simulink model "nmsRR"  (R2021a)
settings: Solver=ode15s  StartTime=0.0  StopTime=t  MaxStep=1e-2  RelTol=1e-2
StartFcn:
  | tic
StopFcn:
  | toc
  | 
  | 
  | %if GimbalLockFlag
  |  % fprintf(2, 'Almost reached Gimbal Lock of IMU. Simulation stopped.\n')
  | %end
  | 
  | %fprintf('Elapsed time: %4.2f sec (%4.2f%% realtime)\n', a, tout(end)/a*100)
undefined symbols (not defined in the file): Balance02, Balance13, BalanceTrunk, BasisStim, CompensateSwing, CompliantLeg, FlexAnkle, Ground, ICs, init_des_left, init_des_right, init_l_left, init_l_right, init_q_del, init_sensor_body, init_sensor_world, init_v_left, init_v_right, LateralControl, mParams, PreventKneeOverextension, StepDur, Target02, Target13, theta0, X, Y, Z
libraries: simulink_extras x133, nesl_utility x105, sm_lib x88, simulink x72, robotcorelib x5, dspinverses x5, dspswit3 x2, vrlib x2, robotmaniplib x1
(part 3 of 8)

== system nmsRR/CMA Data/check steady state ==
  p : Inport
  nStep : Inport  Port=2
  Abs : Abs  ZeroCross=off
  Add{,1..9,15..16} (12 alike) : Sum  Inputs=-+
  Add{10..14,17} (6 alike) : Sum  Inputs=+-
  Demux2 : Demux  Outputs=7
  Demux3 : Demux  Outputs=7
  Fcn : Fcn  Expr=rem(u(1), 2)
  Gain14 : Gain  Gain=.5
  Mux1 : Mux  Inputs=6
  Rounding Function1 : Rounding
  Scope : Scope
  Sum of Elements : Sum  Inputs=+
  even : Subsystem  TreatAsAtomicUnit=on
  odd : Subsystem  TreatAsAtomicUnit=on
  SS_dist : Outport  VectorParamsAs1DForOutWhenUnconnected=off
  wires:
  p/1 -> even/1(In1), odd/1(In1)
  Fcn/1 -> odd/Trigger, even/Trigger
  odd/1(Out1) -> Scope/1, Demux2/1
  even/1(Out1) -> Demux3/1
  Add10/1 -> Mux1/1
  Add11/1 -> Mux1/2
  Add12/1 -> Mux1/3
  Add13/1 -> Mux1/4
  Add14/1 -> Mux1/5
  Demux2/2 -> Add/2
  Demux2/3 -> Add1/2
  Demux2/4 -> Add2/2
  Demux2/5 -> Add3/2
  Demux2/6 -> Add4/2
  Demux2/1 -> Add/1, Add1/1, Add2/1, Add3/1, Add4/1, Add15/1
  Demux3/2 -> Add5/2
  Demux3/3 -> Add6/2
  Demux3/4 -> Add7/2
  Demux3/5 -> Add8/2
  Demux3/6 -> Add9/2
  Demux3/1 -> Add5/1, Add6/1, Add7/1, Add8/1, Add9/1, Add16/1
  Add/1 -> Add10/1
  Add1/1 -> Add11/1
  Add2/1 -> Add12/1
  Add3/1 -> Add13/1
  Add4/1 -> Add14/1
  Add5/1 -> Add10/2
  Add6/1 -> Add11/2
  Add7/1 -> Add12/2
  Add8/1 -> Add13/2
  Add9/1 -> Add14/2
  Mux1/1 -> Abs/1
  Abs/1 -> Sum of Elements/1
  Sum of Elements/1 -> SS_dist/1
  nStep/1 -> Gain14/1
  Gain14/1 -> Rounding Function1/1
  Rounding Function1/1 -> Fcn/1
  Demux2/7 -> Add15/2
  Demux3/7 -> Add16/2
  Add15/1 -> Add17/1
  Add16/1 -> Add17/2
  Add17/1 -> Mux1/6

== system nmsRR/Muscle Actuation Layer/Muscles Left ==
  STIM Left : Inport
  Demux : Demux
  Muscle Dynamics (Vectorized)1 : Subsystem
  Muscle Length Vector1 : Subsystem
  Muscle Torque Contributions1 : Subsystem
  Scope : Scope
  Terminator : Terminator
  Terminator1 : Terminator
  tauHipPitchL : Outport
  tauHipRollL : Outport  Port=2
  tauKneeL : Outport  Port=3
  tauHipAnkleL : Outport  Port=4
  tag scope: LFmVec=global, LLceVec=global, LVceVec=global
  wires:
  Demux/2 -> Muscle Length Vector1/2(qHipRoll [rad])
  Muscle Torque Contributions1/2(tauHR [Nm]) -> tauHipRollL/1
  Demux/1 -> Muscle Length Vector1/1(qHipPitch [rad])
  Muscle Dynamics (Vectorized)1/1(Fmtc) -> Scope/1, Muscle Torque Contributions1/3(FmVec [N x11]), [LFmVec]
  Demux/4 -> Muscle Torque Contributions1/2(qAnkle [rad]), Muscle Length Vector1/4(qAnkle [rad])  "qA"
  Muscle Dynamics (Vectorized)1/3(Vce) -> [LVceVec]
  Muscle Torque Contributions1/3(tauK [Nm]) -> tauKneeL/1
  Demux/3 -> Muscle Torque Contributions1/1(qKnee [rad]), Muscle Length Vector1/3(qKnee [rad])  "qK"
  Muscle Dynamics (Vectorized)1/5(ForceLengthFactor) -> Terminator1/1
  Muscle Length Vector1/1(lmtc [m x11]) -> Muscle Dynamics (Vectorized)1/1(lmtc [m])
  Muscle Torque Contributions1/1(tauHP [Nm]) -> tauHipPitchL/1
  Muscle Torque Contributions1/4(tauA [Nm]) -> tauHipAnkleL/1
  Muscle Dynamics (Vectorized)1/4(A) -> Terminator/1
  Muscle Dynamics (Vectorized)1/2(Lce) -> [LLceVec]
  STIM Left/1 -> Muscle Dynamics (Vectorized)1/2(STIM)
  [Llegq] -> Demux/1

== system nmsRR/Muscle Actuation Layer/Muscles Right ==
  STIM Right : Inport
  Demux : Demux
  Goto15 : Goto  Commented=on  GotoTag=activation_R  TagVisibility=global
  Muscle Dynamics (Vectorized) : Subsystem
  Muscle Length Vector : Subsystem
  Muscle Torque Contributions : Subsystem
  R Leg Muscles Vce [m/s x11]1 : Goto  Commented=on  GotoTag=RForceLength  TagVisibility=global
  tauHipPitchR : Outport
  tauHipRollR : Outport  Port=2
  tauKneeR : Outport  Port=3
  tauHipAnkleR : Outport  Port=4
  tag scope: RFmVec=global, RLceVec=global, RVceVec=global
  wires:
  Muscle Torque Contributions/4(tauA [Nm]) -> tauHipAnkleR/1
  Muscle Torque Contributions/3(tauK [Nm]) -> tauKneeR/1
  Muscle Length Vector/1(lmtc [m x11]) -> Muscle Dynamics (Vectorized)/1(lmtc [m])
  Demux/3 -> Muscle Torque Contributions/1(qKnee [rad]), Muscle Length Vector/3(qKnee [rad])  "qK"
  Demux/4 -> Muscle Torque Contributions/2(qAnkle [rad]), Muscle Length Vector/4(qAnkle [rad])  "qA"
  Muscle Dynamics (Vectorized)/2(Lce) -> [RLceVec]
  Muscle Torque Contributions/2(tauHR [Nm]) -> tauHipRollR/1
  Demux/1 -> Muscle Length Vector/1(qHipPitch [rad])  "qHP"
  Muscle Dynamics (Vectorized)/5(ForceLengthFactor) -> R Leg Muscles Vce [m/s x11]1/1
  Muscle Dynamics (Vectorized)/1(Fmtc) -> Muscle Torque Contributions/3(FmVec [N x11]), [RFmVec]
  Muscle Dynamics (Vectorized)/4(A) -> Goto15/1
  Muscle Dynamics (Vectorized)/3(Vce) -> [RVceVec]
  Muscle Torque Contributions/1(tauHP [Nm]) -> tauHipPitchR/1
  Demux/2 -> Muscle Length Vector/2(qHipRoll [rad])  "qHR"
  STIM Right/1 -> Muscle Dynamics (Vectorized)/2(STIM)
  [Rlegq] -> Demux/1  "qHP"

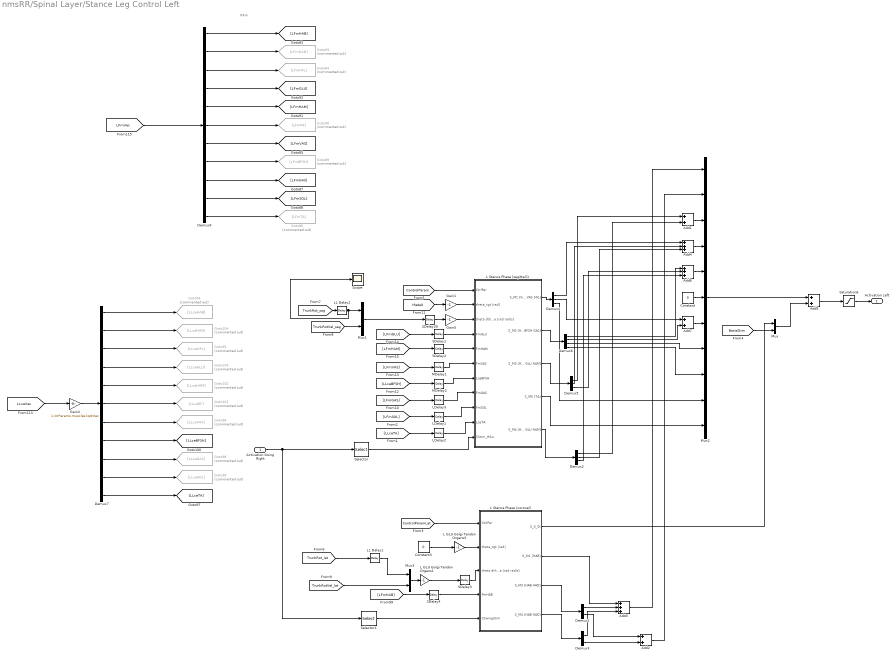
== system nmsRR/Spinal Layer/Stance Leg Control Left ==
  note: RFm
  Activation Swing Right : Inport
  Add{1..2,5,7} (4 alike) : Sum
  Add3 : Sum  Inputs=+++
  Add4 : Sum  Inputs=+++
  Add6 : Sum  Inputs=+++
  Constant : Constant  Value=0
  Constant3 : Constant  Value=0
  Demux1 : Demux  Outputs=2
  Demux2 : Demux  Outputs=3
  Demux3 : Demux  Outputs=2
  Demux4 : Demux  Outputs=3
  Demux5 : Demux  Outputs=3
  Demux6 : Demux
  Demux7 : Demux  Outputs=11
  Demux9 : Demux  Outputs=11
  Gain1 : Gain  Gain=-1
  Gain4 : Gain  Gain=1./mParams.muscles.loptVec
  Gain5 : Gain  Gain=-1
  Goto101 : Goto  Commented=on  GotoTag=LLceRF
  Goto102 : Goto  Commented=on  GotoTag=LLceHAM
  Goto103 : Goto  Commented=on  GotoTag=LLceGLU
  Goto104 : Goto  Commented=on  GotoTag=LLceHAD
  Goto84 : Goto  Commented=on  GotoTag=LFmHFL
  Goto86 : Goto  Commented=on  GotoTag=LFmTA
  Goto89 : Goto  Commented=on  GotoTag=LFmBFSH
  Goto90 : Goto  Commented=on  GotoTag=LFmRF
  Goto93 : Goto  Commented=on  GotoTag=LFmHAD
  Goto94 : Goto  Commented=on  GotoTag=LLceHAB
  Goto95 : Goto  Commented=on  GotoTag=LLceHFL
  Goto96 : Goto  Commented=on  GotoTag=LLceVAS
  Goto98 : Goto  Commented=on  GotoTag=LLceGAS
  Goto99 : Goto  Commented=on  GotoTag=LLceSOL
  L GLU Golgi Tendon Organs1 : Gain  Gain=-1
  L GLU Golgi Tendon Organs3 : Gain  Gain=-1
  L Stance Phase (coronal) : Subsystem  TreatAsAtomicUnit=on
  L Stance Phase (sagittal)1 : Subsystem  TreatAsAtomicUnit=on
  LDelay1 : TransportDelay  DelayTime=mParams.control.delays.long
  LDelay2 : TransportDelay  DelayTime=mParams.control.delays.long
  LDelay3 : TransportDelay  DelayTime=mParams.control.delays.long
  LL Delay1 : TransportDelay  DelayTime=mParams.control.delays.longloop/2
  LL Delay2 : TransportDelay  DelayTime=mParams.control.delays.longloop/2
  MDelay1 : TransportDelay  DelayTime=mParams.control.delays.mid
  MDelay2 : TransportDelay  DelayTime=mParams.control.delays.mid
  Mux : Mux  Inputs=2
  Mux1 : Mux  Inputs=2
  Mux2 : Mux  Inputs=11
  Mux3 : Mux  Inputs=2
  SDelay{1..4,29} (5 alike) : TransportDelay  DelayTime=mParams.control.delays.short
  Saturation6 : Saturate  UpperLimit=1  LowerLimit=0.01  ZeroCross=off
  Scope : Scope
  Selector : Selector  InputPortWidth=11  IndexOptions=Index vector (dialog)  Indices=[3 4 5 6]  OutputSizes=1
  Selector1 : Selector  InputPortWidth=11  IndexOptions=Index vector (dialog)  Indices=[1 2]  OutputSizes=1
  Activation Left : Outport
  wires:
  [LFmVec] -> Demux9/1
  Demux9/1 -> [LFmHAB]
  [ControlParam] -> L Stance Phase (sagittal)1/1(CtrlPar)
  Demux7/5 -> Goto102/1
  MDelay1/1 -> L Stance Phase (sagittal)1/6(FmVAS)
  Gain4/1 -> Demux7/1
  Demux9/5 -> [LFmHAM]
  Demux7/10 -> Goto99/1
  Demux7/8 -> [LLceBFSH]
  Mux1/1 -> SDelay29/1
  Demux7/3 -> Goto95/1
  Demux7/9 -> Goto98/1
  LDelay2/1 -> L Stance Phase (sagittal)1/10(LceTA)
  Demux9/3 -> Goto84/1
  LDelay1/1 -> L Stance Phase (sagittal)1/9(FmSOL)
  Demux9/11 -> Goto86/1
  [LLceVec] -> Gain4/1
  Demux9/9 -> [LFmGAS]
  Demux7/4 -> Goto103/1
  SDelay2/1 -> L Stance Phase (sagittal)1/5(FmHAM)
  Demux9/10 -> [LFmSOL]
  Gain5/1 -> L Stance Phase (sagittal)1/3(theta dtheta [rad rad/s])
  Demux7/2 -> Goto104/1
  Demux9/4 -> [LFmGLU]
  SDelay29/1 -> Gain5/1
  Demux9/6 -> Goto90/1
  Demux9/8 -> Goto89/1
  Demux9/7 -> [LFmVAS]
  Demux7/11 -> [LLceTA]
  LDelay3/1 -> L Stance Phase (sagittal)1/8(FmGAS)
  SDelay1/1 -> L Stance Phase (sagittal)1/4(FmGLU)
  Demux7/7 -> Goto96/1
  Demux7/1 -> Goto94/1
  Demux9/2 -> Goto93/1
  Demux7/6 -> Goto101/1
  MDelay2/1 -> L Stance Phase (sagittal)1/7(LceBFSH)
  Saturation6/1 -> Activation Left/1
  Add5/1 -> Saturation6/1
  Mux/1 -> Add5/2
  [theta0] -> Gain1/1
  Gain1/1 -> L Stance Phase (sagittal)1/2(theta_tgt [rad])
  [BasisStim] -> Mux/2
  [ControlParamLat] -> L Stance Phase (coronal)/1(CtrlPar)
  SDelay3/1 -> L Stance Phase (coronal)/3(theta dtheta [rad rad/s])
  [LFmHAB] -> SDelay4/1
  SDelay4/1 -> L Stance Phase (coronal)/4(FmHAB)
  L GLU Golgi Tendon Organs1/1 -> SDelay3/1
  L GLU Golgi Tendon Organs3/1 -> L Stance Phase (coronal)/2(theta_tgt [rad])
  Constant3/1 -> L GLU Golgi Tendon Organs3/1
  Mux3/1 -> L GLU Golgi Tendon Organs1/1
  L Stance Phase (coronal)/1(S_0_St) -> Mux/1
  L Stance Phase (coronal)/2(S_M1 [HAB]) -> Add3/1
  L Stance Phase (coronal)/3(S_M3 [HAB HAD]) -> Demux1/1
  Demux1/1 -> Add3/2
  [TrunkRot_sag] -> LL Delay2/1
  LL Delay2/1 -> Scope/1, Mux1/1
  [TrunkRotVel_sag] -> Mux1/2
  [TrunkRot_lat] -> LL Delay1/1
  LL Delay1/1 -> Mux3/1
  [TrunkRotVel_lat] -> Mux3/2
  [LFmGLU] -> SDelay1/1
  [LFmHAM] -> SDelay2/1
  [LFmVAS] -> MDelay1/1
  [LLceBFSH] -> MDelay2/1
  [LFmGAS] -> LDelay3/1
  [LFmSOL] -> LDelay1/1
  [LLceTA] -> LDelay2/1
  Demux4/3 -> Mux2/10
  Constant/1 -> Mux2/6
  L Stance Phase (sagittal)1/2(S_M2 [HAM VAS BFSH GAS]) -> Demux6/1
  Add6/1 -> Mux2/5
  Demux6/2 -> Add7/2
  Add4/1 -> Mux2/4
  Demux4/1 -> Add4/1
  Add3/1 -> Mux2/1
  Demux4/2 -> Add7/1
  Demux6/4 -> Mux2/9
  L Stance Phase (sagittal)1/4(S_M5 [TA]) -> Mux2/11
  Demux1/2 -> Add2/1
  Demux6/3 -> Mux2/8
  Mux2/1 -> Add5/1
  Add7/1 -> Mux2/7
  Demux6/1 -> Add6/1
  Demux5/1 -> Add1/1
  Demux5/2 -> Add4/2
  Demux5/3 -> Add6/2
  L Stance Phase (sagittal)1/1(S_M1 [GLU VAS SOL]) -> Demux4/1
  L Stance Phase (sagittal)1/3(S_M3 [HFL GLU HAM]) -> Demux5/1
  Selector/1 -> L Stance Phase (sagittal)1/11(CStim_HSw)
  L Stance Phase (sagittal)1/5(S_M4 [HFL GLU HAM]) -> Demux2/1
  Add1/1 -> Mux2/3
  Demux2/1 -> Add1/2
  Demux2/2 -> Add4/3
  Demux2/3 -> Add6/3
  L Stance Phase (coronal)/4(S_M4 [HAB HAD]) -> Demux3/1
  Demux3/1 -> Add3/3
  Demux3/2 -> Add2/2
  Add2/1 -> Mux2/2
  Activation Swing Right/1 -> Selector1/1, Selector/1
  Selector1/1 -> L Stance Phase (coronal)/5(CSwingStim)

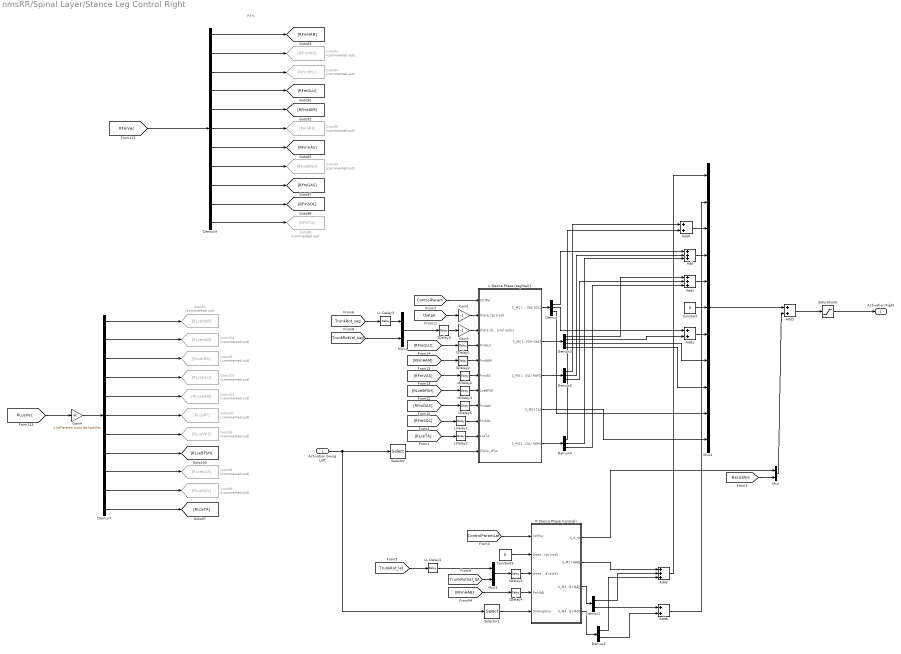
== system nmsRR/Spinal Layer/Stance Leg Control Right ==
  note: RFm
  Activation Swing Left : Inport
  Add : Sum  Inputs=+++
  Add1 : Sum  Inputs=+++
  Add{2,4..6} (4 alike) : Sum
  Add3 : Sum  Inputs=+++
  Constant : Constant  Value=0
  Constant3 : Constant  Value=0
  Demux : Demux  Outputs=3
  Demux1 : Demux  Outputs=2
  Demux2 : Demux  Outputs=3
  Demux3 : Demux
  Demux4 : Demux  Outputs=3
  Demux5 : Demux  Outputs=2
  Demux7 : Demux  Outputs=11
  Demux9 : Demux  Outputs=11
  Gain1 : Gain  Gain=-1
  Gain4 : Gain  Gain=1./mParams.muscles.loptVec
  Gain5 : Gain  Gain=-1
  Goto101 : Goto  Commented=on  GotoTag=RLceRF
  Goto102 : Goto  Commented=on  GotoTag=RLceHAM
  Goto103 : Goto  Commented=on  GotoTag=RLceGLU
  Goto104 : Goto  Commented=on  GotoTag=RLceHAD
  Goto84 : Goto  Commented=on  GotoTag=RFmHFL
  Goto86 : Goto  Commented=on  GotoTag=RFmTA
  Goto89 : Goto  Commented=on  GotoTag=RFmBFSH
  Goto90 : Goto  Commented=on  GotoTag=RFmRF
  Goto93 : Goto  Commented=on  GotoTag=RFmHAD
  Goto94 : Goto  Commented=on  GotoTag=RLceHAB
  Goto95 : Goto  Commented=on  GotoTag=RLceHFL
  Goto96 : Goto  Commented=on  GotoTag=RLceVAS
  Goto98 : Goto  Commented=on  GotoTag=RLceGAS
  Goto99 : Goto  Commented=on  GotoTag=RLceSOL
  L Stance Phase (sagittal)1 : Subsystem  TreatAsAtomicUnit=on
  LDelay1 : TransportDelay  DelayTime=mParams.control.delays.long
  LDelay2 : TransportDelay  DelayTime=mParams.control.delays.long
  LDelay6 : TransportDelay  DelayTime=mParams.control.delays.long
  LL Delay1 : TransportDelay  DelayTime=mParams.control.delays.longloop/2
  LL Delay3 : TransportDelay  DelayTime=mParams.control.delays.longloop/2
  MDelay2 : TransportDelay  DelayTime=mParams.control.delays.mid
  MDelay3 : TransportDelay  DelayTime=mParams.control.delays.mid
  Mux : Mux  Inputs=2
  Mux1 : Mux  Inputs=2
  Mux3 : Mux  Inputs=2
  Mux4 : Mux  Inputs=11
  R Stance Phase (coronal) : Subsystem  TreatAsAtomicUnit=on
  SDelay{1..5} (5 alike) : TransportDelay  DelayTime=mParams.control.delays.short
  Saturation6 : Saturate  UpperLimit=1  LowerLimit=0.01  ZeroCross=off
  Selector : Selector  InputPortWidth=11  IndexOptions=Index vector (dialog)  Indices=[3 4 5 6]  OutputSizes=1
  Selector1 : Selector  InputPortWidth=11  IndexOptions=Index vector (dialog)  Indices=[1 2]  OutputSizes=1
  Activation Right : Outport
  wires:
  [RFmVec] -> Demux9/1
  Demux9/1 -> [RFmHAB]
  [ControlParam] -> L Stance Phase (sagittal)1/1(CtrlPar)
  Demux7/5 -> Goto102/1
  Add/1 -> Mux4/4
  MDelay2/1 -> L Stance Phase (sagittal)1/6(FmVAS)
  Gain4/1 -> Demux7/1
  Demux9/5 -> [RFmHAM]
  Demux7/10 -> Goto99/1
  Demux7/8 -> [RLceBFSH]
  Mux1/1 -> SDelay3/1
  Demux7/3 -> Goto95/1
  Demux7/9 -> Goto98/1
  LDelay2/1 -> L Stance Phase (sagittal)1/10(LceTA)
  Demux9/3 -> Goto84/1
  LDelay1/1 -> L Stance Phase (sagittal)1/9(FmSOL)
  Mux4/1 -> Add5/1
  Demux9/11 -> Goto86/1
  Demux9/9 -> [RFmGAS]
  Demux7/4 -> Goto103/1
  SDelay2/1 -> L Stance Phase (sagittal)1/5(FmHAM)
  Demux9/10 -> [RFmSOL]
  Gain5/1 -> L Stance Phase (sagittal)1/3(theta dtheta [rad rad/s])
  Demux7/2 -> Goto104/1
  Demux9/4 -> [RFmGLU]
  SDelay3/1 -> Gain5/1
  Demux9/6 -> Goto90/1
  Demux9/8 -> Goto89/1
  Demux9/7 -> [RFmVAS]
  Demux7/11 -> [RLceTA]
  LDelay6/1 -> L Stance Phase (sagittal)1/8(FmGAS)
  SDelay1/1 -> L Stance Phase (sagittal)1/4(FmGLU)
  Demux7/7 -> Goto96/1
  Demux7/1 -> Goto94/1
  Demux9/2 -> Goto93/1
  Demux7/6 -> Goto101/1
  Add2/1 -> Mux4/7
  MDelay3/1 -> L Stance Phase (sagittal)1/7(LceBFSH)
  L Stance Phase (sagittal)1/2(S_M2 [HAM VAS BFSH GAS]) -> Demux3/1
  Add1/1 -> Mux4/5
  Demux/1 -> Add/1
  Demux/2 -> Add2/1
  Demux/3 -> Mux4/10
  Demux3/1 -> Add1/1
  Demux3/2 -> Add2/2
  Demux3/4 -> Mux4/9
  Demux2/1 -> Add4/1
  Demux2/2 -> Add/2
  Demux2/3 -> Add1/2
  [BasisStim] -> Mux/2
  Saturation6/1 -> Activation Right/1
  Add5/1 -> Saturation6/1
  [RLceVec] -> Gain4/1
  L Stance Phase (sagittal)1/1(S_M1 [GLU VAS SOL]) -> Demux/1
  [theta0] -> Gain1/1
  L Stance Phase (sagittal)1/4(S_M5 [TA]) -> Mux4/11
  Gain1/1 -> L Stance Phase (sagittal)1/2(theta_tgt [rad])
  L Stance Phase (sagittal)1/3(S_M3 [HFL GLU HAM]) -> Demux2/1
  R Stance Phase (coronal)/1(S_0_St) -> Mux/1
  Constant3/1 -> R Stance Phase (coronal)/2(theta_tgt [rad])
  SDelay5/1 -> R Stance Phase (coronal)/3(theta dtheta [rad rad/s])
  [RFmHAB] -> SDelay4/1
  [ControlParamLat] -> R Stance Phase (coronal)/1(CtrlPar)
  SDelay4/1 -> R Stance Phase (coronal)/4(FmHAB)
  Mux3/1 -> SDelay5/1
  Mux/1 -> Add5/2
  R Stance Phase (coronal)/3(S_M3 [HAB HAD]) -> Demux1/1
  R Stance Phase (coronal)/2(S_M1 [HAB]) -> Add3/1
  Demux1/1 -> Add3/2
  Add3/1 -> Mux4/1
  Demux1/2 -> Add6/1
  [TrunkRotVel_lat] -> Mux3/2
  [TrunkRot_sag] -> LL Delay3/1
  Demux3/3 -> Mux4/8
  LL Delay3/1 -> Mux1/1
  [TrunkRotVel_sag] -> Mux1/2
  [TrunkRot_lat] -> LL Delay1/1
  LL Delay1/1 -> Mux3/1
  Constant/1 -> Mux4/6
  [RLceTA] -> LDelay2/1
  [RFmSOL] -> LDelay1/1
  [RFmGAS] -> LDelay6/1
  [RLceBFSH] -> MDelay3/1
  [RFmVAS] -> MDelay2/1
  [RFmGLU] -> SDelay1/1
  [RFmHAM] -> SDelay2/1
  Selector/1 -> L Stance Phase (sagittal)1/11(CStim_HSw)
  L Stance Phase (sagittal)1/5(S_M4 [HFL GLU HAM]) -> Demux4/1
  Add4/1 -> Mux4/3
  Demux4/1 -> Add4/2
  Demux4/2 -> Add/3
  Demux4/3 -> Add1/3
  Activation Swing Left/1 -> Selector1/1, Selector/1
  Selector1/1 -> R Stance Phase (coronal)/5(CSwingStim)
  R Stance Phase (coronal)/4(S_M4 [HAB HAD]) -> Demux5/1
  Demux5/2 -> Add6/2
  Demux5/1 -> Add3/3
  Add6/1 -> Mux4/2

== system nmsRR/Spinal Layer/Stretch Reflex for Swing Leg Control ==
  note: sensor time delay low-pass filter
  note: input: descending commands
  note: stretch reflex
  note: saturation
  note: output: STIM
  Descending Commands Left : Inport
  Descending Commands Right : Inport  Port=2
  LPF 11x0.0025s : Subsystem
  LPF 11x0.0025s1 : Subsystem
  LPF 11x0.0025s2 : Subsystem
  LPF 11x0.0025s3 : Subsystem
  LPF 11x0.0025s4 : Subsystem
  LPF 11x0.0025s5 : Subsystem
  LPF 11x0.0025s6 : Subsystem
  LPF 11x0.0025s7 : Subsystem
  Saturation4 : Saturate  UpperLimit=1  LowerLimit=0.001  ZeroCross=off
  Saturation6 : Saturate  UpperLimit=1  LowerLimit=0.001  ZeroCross=off
  Stretch Reflex Left : Subsystem
  Stretch Reflex Right : Subsystem
  Activation Left : Outport
  Activation Right : Outport  Port=2
  wires:
  Descending Commands Left/1 -> LPF 11x0.0025s5/1(in), LPF 11x0.0025s/1(in)
  Descending Commands Right/1 -> LPF 11x0.0025s3/1(in), LPF 11x0.0025s7/1(in)
  Saturation4/1 -> Activation Right/1
  Saturation6/1 -> Activation Left/1
  Stretch Reflex Left/1(STIM) -> Saturation6/1
  Stretch Reflex Right/1(STIM) -> Saturation4/1
  [LLceVec] -> LPF 11x0.0025s1/1(in)
  [LVceVec] -> LPF 11x0.0025s2/1(in)
  [RLceVec] -> LPF 11x0.0025s4/1(in)
  LPF 11x0.0025s1/1(l) -> Stretch Reflex Left/3(l_ce)
  LPF 11x0.0025s6/1(v) -> Stretch Reflex Right/4(v_ce)
  LPF 11x0.0025s2/1(v) -> Stretch Reflex Left/4(v_ce)
  LPF 11x0.0025s/1(lambda) -> Stretch Reflex Left/1(lambda)
  LPF 11x0.0025s3/1(lambda) -> Stretch Reflex Right/1(lambda)
  LPF 11x0.0025s4/1(l) -> Stretch Reflex Right/3(l_ce)
  [RVceVec] -> LPF 11x0.0025s6/1(in)
  LPF 11x0.0025s5/1(lambda dot) -> Stretch Reflex Left/2(lambda_dot)
  LPF 11x0.0025s7/1(lambda dot) -> Stretch Reflex Right/2(lambda_dot)

== system nmsRR/Supraspinal Level/Finite State Machine ==
  note: Finite State Machine (FSM): The FSM comprises 4 states (Early Right Swing (0), Late Right Swing (1), Early Left Swing (2) and Late Left Swing (3)). The FSM transitions from state 0 to state 1 and from state 2 to state 3 when the time dt in state 0/2 is passed. It transitions from state 2 to state 3 and from state 3 to state 1 when right/left contact is measured.
  Information: Ground Contact : Inport
  Chart : Stateflow chart  TreatAsAtomicUnit=on
  Constant : Constant  Value=StepDur*0.6
  Demux : Demux  Outputs=2
  Early Right Swing : Outport
  Late Right Swing : Outport  Port=2
  Early Left Swing : Outport  Port=3
  Late Left Swing : Outport  Port=4
  wires:
  Demux/1 -> Chart/2(contact_left)
  Constant/1 -> Chart/1(dt)
  Demux/2 -> Chart/3(contact_right)
  Information: Ground Contact/1 -> Demux/1
  Chart/1(state0) -> Early Right Swing/1
  Chart/2(state1) -> Late Right Swing/1
  Chart/3(state2) -> Early Left Swing/1
  Chart/4(state3) -> Late Left Swing/1

== system nmsRR/Supraspinal Level/Subsystem ==
  note: Goal State
  note: Movement Plan
  note: Inverse Dynamics
  note: Moment Arm Inversion
  note: Invert Muscle Dynamics
  note: Invert Stretch Reflex
  note: input: behavioral states
  note: output: descending commands
  Early/Late Swing : Inport
  Left/Right : Inport  Port=2
  Compute Acceleration Profiles with Minimal Jerk Approach : Subsystem
  Compute Target States : Subsystem
  Inverse Dynamics : Subsystem
  Inversion of Muscle Model : Subsystem
  Mux : Mux
  Stretch Reflex Inversion : Subsystem
  Terminator : Terminator
  To Workspace1 : ToWorkspace  VariableName=DesiredAccelerations  SampleTime=-1
      settings: Save2DSignal=2-D array (concatenate along first dimension)
  To Workspace3 : ToWorkspace  VariableName=TargetStates  SampleTime=-1
      settings: Save2DSignal=2-D array (concatenate along first dimension)
  torques --> forces : Subsystem
  Descending Command Left : Outport
  Descending Command Right : Outport  Port=2
  Desired Torques : Outport  Port=3
  wires:
  Inverse Dynamics/1(Desired Torques) -> Desired Torques/1, torques --> forces/1(Desired Torque)
  Compute Target States/3(Ankle Target) -> Compute Acceleration Profiles with Minimal Jerk Approach/3(Target State Ankle), Mux/3
  Compute Target States/4(Hip Roll Target) -> Compute Acceleration Profiles with Minimal Jerk Approach/4(Target State Hip Roll), Mux/4
  Left/Right/1 -> Compute Acceleration Profiles with Minimal Jerk Approach/5(Swing Right/Left), Compute Target States/1(Left/Right)
  Stretch Reflex Inversion/2(Descending Command Right) -> Descending Command Right/1
  Compute Target States/2(Knee Target) -> Compute Acceleration Profiles with Minimal Jerk Approach/2(Target State Knee), Mux/2
  Compute Target States/1(Hip Pitch Target) -> Compute Acceleration Profiles with Minimal Jerk Approach/1(Target State Hip Pitch), Mux/1
  Inversion of Muscle Model/1(Desired Activation Left) -> Stretch Reflex Inversion/1(Desired Activation Left)
  Compute Acceleration Profiles with Minimal Jerk Approach/1("Desired Acceleration ") -> To Workspace1/1, Inverse Dynamics/1(Desired Acceleration)
  Stretch Reflex Inversion/1(Descending Command Left) -> Descending Command Left/1
  Inversion of Muscle Model/2(Desired Activation Right) -> Stretch Reflex Inversion/2(Desired Activation Right)
  Early/Late Swing/1 -> Compute Target States/2(Early/Late Swing), Compute Acceleration Profiles with Minimal Jerk Approach/6(Early/Late Swing)
  Mux/1 -> To Workspace3/1
  Compute Acceleration Profiles with Minimal Jerk Approach/2(Joint Angles Swing) -> Terminator/1
  torques --> forces/1(Desired Force) -> Inversion of Muscle Model/1(Desired Forces)

== system nmsRR/Body and Contact Model/L Leg/Ankle Mechanical Limits ==
  note: Overextension Torque
  note: Joint Limits
  note: Overflexion Torque
  dq [rad/s] : Inport
  q [rad] : Inport  Port=2
  Gain1 : Gain  Gain=mParams.joints.ankle.kStop
  Gain2 : Gain  Gain=-1
  Gain3 : Gain  Gain=mParams.joints.ankle.kStop
  Gain4 : Gain  Gain=1/mParams.joints.ankle.wMaxStop
  Gain5 : Gain  Gain=-1
  Gain6 : Gain  Gain=-1
  Limit Knee Range : simulink/Logic and Bit Operations/Interval Test  Commented=on  IntervalClosedRight=on  uplimit=mParams.joints.ankle.MaxPitch + 20*pi/180  IntervalClosedLeft=on  lowlimit=mParams.joints.ankle.MinPitch - 20*pi/180  OutDataTypeStr=boolean
      settings: AttributesFormatString=|
      | Lower limits: %<lowlimit>
      | Upper limits: %<uplimit>
  Logical Operator3 : Logic  Commented=on  Operator=NOT  AllPortsSameDT=off  OutDataTypeStr=boolean
  Product1 : Product  Inputs=4
  Product2 : Product  Inputs=4
  Stop Simulation1 : Stop  Commented=on
  Sum : Sum  Inputs=|+-
  Sum1 : Sum  Inputs=|+-
  Sum2 : Sum
  Sum3 : Sum  Inputs=|-+
  Sum4 : Sum  Inputs=|-+
  above upper limit? : simulink/Logic and Bit Operations/Compare To Zero  relop=>  OutDataTypeStr=boolean  ZeroCross=off
  below lower limit? : simulink/Logic and Bit Operations/Compare To Zero  relop=<  OutDataTypeStr=boolean  ZeroCross=off
  const : Constant
  const1 : Constant
  mech limit pushes back? : simulink/Logic and Bit Operations/Compare To Zero  relop=>  OutDataTypeStr=boolean  ZeroCross=off
  mech limit pushes back?. : simulink/Logic and Bit Operations/Compare To Zero  relop=>  OutDataTypeStr=boolean  ZeroCross=off
  overextension angle : Constant  Value=mParams.joints.ankle.MaxPitch
  overflexion angle : Constant  Value=mParams.joints.ankle.MinPitch
  tau [Nm] : Outport  VectorParamsAs1DForOutWhenUnconnected=off
  wires:
  Logical Operator3/1 -> Stop Simulation1/1
  Limit Knee Range/1 -> Logical Operator3/1
  Gain6/1 -> Sum2/1
  Gain2/1 -> Sum3/1
  Sum2/1 -> tau [Nm]/1
  overflexion angle/1 -> Sum1/2
  Sum1/1 -> Gain1/1
  Sum/1 -> Gain3/1
  q [rad]/1 -> Sum1/1, Limit Knee Range/1, Sum/1
  overextension angle/1 -> Sum/2
  dq [rad/s]/1 -> Gain4/1
  const/1 -> Sum3/2
  Sum3/1 -> Product1/3, mech limit pushes back?/1
  Gain3/1 -> Product1/2, above upper limit?/1
  mech limit pushes back?/1 -> Product1/4
  above upper limit?/1 -> Product1/1
  Product1/1 -> Gain6/1
  Product2/1 -> Gain5/1
  below lower limit?/1 -> Product2/1
  mech limit pushes back?./1 -> Product2/4
  Gain1/1 -> below lower limit?/1, Product2/2
  Sum4/1 -> mech limit pushes back?./1, Product2/3
  const1/1 -> Sum4/2
  Gain4/1 -> Sum4/1, Gain2/1
  Gain5/1 -> Sum2/2

== system nmsRR/Body and Contact Model/L Leg/Foot ==
  "  XYZ Sensor Ball left" : Subsystem
  B Transform : sm_lib/Frames and Transforms/Rigid Transform  TranslationMethod=Cartesian  TranslationStandardOffset=0  TranslationLengthUnit=m  TranslationStandardAxis=+Y  TranslationCartesianOffset=[ mParams.bodies.foot.compensation mParams.bodies.foot.l/2 0]  TranslationROffset=0  TranslationROffsetUnits=m  TranslationZOffset=0  TranslationZOffsetUnits=m  TranslationThetaOffset=0  TranslationThetaOffsetUnits=deg  RotationMethod=None  RotationAngleUnits=deg  RotationStandardAxis=+X  RotationAngle=90  RotationArbitraryAxis=[0 0 1]  FollAlignAxisA=+X  BaseAlignAxisA=+Y  FollAlignAxisB=+Y  BaseAlignAxisB=+Z  RotationSequenceAxes=FollowerAxes  RotationSequence=XYX  RotationSequenceAngles=[0 0 0]  RotationSequenceAnglesUnits=deg  RotationMatrix=[1 0 0; 0 1 0; 0 0 1]
  LB Transform : sm_lib/Frames and Transforms/Rigid Transform  TranslationMethod=Cartesian  TranslationStandardOffset=0  TranslationLengthUnit=m  TranslationStandardAxis=+Y  TranslationCartesianOffset="[mParams.bodies.foot.l/2 -mParams.bodies.foot.compensation  -mParams.bodies.foot.BallWidth/2]"  TranslationROffset=0  TranslationROffsetUnits=m  TranslationZOffset=0  TranslationZOffsetUnits=m  TranslationThetaOffset=0  TranslationThetaOffsetUnits=deg  RotationMethod=None  RotationAngleUnits=deg  RotationStandardAxis=+X  RotationAngle=90  RotationArbitraryAxis=[0 0 1]  FollAlignAxisA=+X  BaseAlignAxisA=+Y  FollAlignAxisB=+Y  BaseAlignAxisB=+Z  RotationSequenceAxes=FollowerAxes  RotationSequence=XYX  RotationSequenceAngles=[0 0 0]  RotationSequenceAnglesUnits=deg  RotationMatrix=[1 0 0; 0 1 0; 0 0 1]
  LH Transform : sm_lib/Frames and Transforms/Rigid Transform  TranslationMethod=Cartesian  TranslationStandardOffset=0  TranslationLengthUnit=m  TranslationStandardAxis=+Y  TranslationCartesianOffset="[-mParams.bodies.foot.l/2 -mParams.bodies.foot.compensation  -mParams.bodies.foot.HeelWidth/2]"  TranslationROffset=0  TranslationROffsetUnits=m  TranslationZOffset=0  TranslationZOffsetUnits=m  TranslationThetaOffset=0  TranslationThetaOffsetUnits=deg  RotationMethod=None  RotationAngleUnits=deg  RotationStandardAxis=+X  RotationAngle=90  RotationArbitraryAxis=[0 0 1]  FollAlignAxisA=+X  BaseAlignAxisA=+Y  FollAlignAxisB=+Y  BaseAlignAxisB=+Z  RotationSequenceAxes=FollowerAxes  RotationSequence=XYX  RotationSequenceAngles=[0 0 0]  RotationSequenceAnglesUnits=deg  RotationMatrix=[1 0 0; 0 1 0; 0 0 1]
  RB Transform : sm_lib/Frames and Transforms/Rigid Transform  TranslationMethod=Cartesian  TranslationStandardOffset=0  TranslationLengthUnit=m  TranslationStandardAxis=+Z  TranslationCartesianOffset="[mParams.bodies.foot.l/2 -mParams.bodies.foot.compensation  mParams.bodies.foot.BallWidth/2]"  TranslationROffset=0  TranslationROffsetUnits=m  TranslationZOffset=0  TranslationZOffsetUnits=m  TranslationThetaOffset=0  TranslationThetaOffsetUnits=deg  RotationMethod=None  RotationAngleUnits=deg  RotationStandardAxis=+Z  RotationAngle=0.0  RotationArbitraryAxis=[0 0 1]  FollAlignAxisA=+X  BaseAlignAxisA=+Y  FollAlignAxisB=+Y  BaseAlignAxisB=+Z  RotationSequenceAxes=FollowerAxes  RotationSequence=XYX  RotationSequenceAngles=[0 0 0]  RotationSequenceAnglesUnits=deg  RotationMatrix=[1 0 0; 0 1 0; 0 0 1]
  RH Transform : sm_lib/Frames and Transforms/Rigid Transform  TranslationMethod=Cartesian  TranslationStandardOffset=0  TranslationLengthUnit=m  TranslationStandardAxis=+Z  TranslationCartesianOffset="[-mParams.bodies.foot.l/2 -mParams.bodies.foot.compensation  mParams.bodies.foot.HeelWidth/2]"  TranslationROffset=0  TranslationROffsetUnits=m  TranslationZOffset=0  TranslationZOffsetUnits=m  TranslationThetaOffset=0  TranslationThetaOffsetUnits=deg  RotationMethod=None  RotationAngleUnits=deg  RotationStandardAxis=+Z  RotationAngle=0.0  RotationArbitraryAxis=[0 0 1]  FollAlignAxisA=+X  BaseAlignAxisA=+Y  FollAlignAxisB=+Y  BaseAlignAxisB=+Z  RotationSequenceAxes=FollowerAxes  RotationSequence=XYX  RotationSequenceAngles=[0 0 0]  RotationSequenceAnglesUnits=deg  RotationMatrix=[1 0 0; 0 1 0; 0 0 1]
  Solid1 : sm_lib/Body Elements/Brick Solid  GraphicAmbientColor=[0.15 0.15 0.15 1.0]  BasedOnType=Density  BrickDimensions="[mParams.bodies.foot.l  mParams.bodies.foot.d mParams.bodies.foot.b]"  BrickDimensionUnits=m  CenterOfMass=mParams.bodies.foot.CG  CenterOfMassUnits=m  GraphicDiffuseColor=[1 0.5 0.5]  Density=2.7  DensityUnits=g/cm^3  DoExposeReferenceFrame=on  GraphicEmissiveColor=[0 0 0 1.0]  ExportEntireGeometry=off  SerializedFrames=<Frames><Frame><Id>Frame1</Id><Value><Name>CG</Name><Origin><Source>CenterOfMassFrame</Source><FeatureName></FeatureName></Origin><PrimaryAxis><DefinedDirection>+Z</DefinedDirection><Source>ReferenceFrame</Source><SourceDirection>+Z</SourceDirection><FeatureName></FeatureName></PrimaryAxis><SecondaryAxis><DefinedDirection>+X</DefinedDirection><Source>ReferenceFrame</Source><SourceDirection>+X</SourceDirection><FeatureName></FeatureName></SecondaryAxis></Value></Frame></Frames>  MarkerShape=Sphere  MarkerSize=10  GraphicType=FromGeometry  InertiaType=Custom  Mass=mParams.bodies.foot.m  MassUnits=kg  MomentsOfInertia=mParams.bodies.foot.In  MomentsOfInertiaUnits=kg*m^2  GraphicOpacity=1.0  ProductsOfInertia=[0 0 0]  ProductsOfInertiaUnits=kg*m^2  GraphicShininess=75  GraphicSpecularColor=[0.5 0.5 0.5 1.0]  GraphicVisPropType=SimpleVisualProperties
  Terminator2 : Terminator
  To Workspace4 : ToWorkspace  VariableName=Ball_left  SampleTime=-1
      settings: Save2DSignal=2-D array (concatenate along first dimension)
  Transform CS1(Ankle) to MidSegment1 : sm_lib/Frames and Transforms/Rigid Transform  TranslationMethod=Cartesian  TranslationStandardOffset=0  TranslationLengthUnit=m  TranslationStandardAxis=+Y  TranslationCartesianOffset=mParams.bodies.foot.AnkleToMid  TranslationROffset=0  TranslationROffsetUnits=m  TranslationZOffset=0  TranslationZOffsetUnits=m  TranslationThetaOffset=0  TranslationThetaOffsetUnits=deg  RotationMethod=RotationSequence  RotationAngleUnits=deg  RotationStandardAxis=+X  RotationAngle=-90  RotationArbitraryAxis=[0 0 1]  FollAlignAxisA=+X  BaseAlignAxisA=+Y  FollAlignAxisB=+Y  BaseAlignAxisB=+Z  RotationSequenceAxes=FollowerAxes  RotationSequence=ZXY  RotationSequenceAngles=[90 0 0]  RotationSequenceAnglesUnits=deg  RotationMatrix=[1 0 0; 0 1 0; 0 0 1]
  CS1 : PMIOPort  Side=Left
  Left Ball : PMIOPort  Port=2  Side=Right
  Left Heel : PMIOPort  Port=3  Side=Left
  Right Ball : PMIOPort  Port=4  Side=Right
  Right Heel : PMIOPort  Port=5  Side=Left
  tag scope: Ball_left=global
  wires:
  "  XYZ Sensor Ball left"/2(v_bLH [m/s x3]) -> Terminator2/1
  "  XYZ Sensor Ball left"/1(p_bLH [m x3]) -> To Workspace4/1, [Ball_left]
  connections:
  Transform CS1(Ankle) to MidSegment1/RConn1 -- Solid1/RConn1 -- RB Transform/LConn1 -- RH Transform/LConn1 -- B Transform/LConn1 -- LH Transform/LConn1 -- LB Transform/LConn1
  Transform CS1(Ankle) to MidSegment1/LConn1 -- CS1/RConn1
  Left Heel/RConn1 -- LH Transform/RConn1
  Left Ball/RConn1 -- LB Transform/RConn1
  Right Heel/RConn1 -- RH Transform/RConn1
  Right Ball/RConn1 -- RB Transform/RConn1
  B Transform/RConn1 -- "  XYZ Sensor Ball left"/LConn1

== system nmsRR/Body and Contact Model/L Leg/Hip Pitch Mechanical Limits ==
  note: Overflexion Torque
  note: Joint Limits
  note: Overextension Torque
  dq [rad/s] : Inport
  q [rad] : Inport  Port=2
  Gain1 : Gain  Gain=mParams.joints.hip.kStop
  Gain2 : Gain  Gain=-1
  Gain3 : Gain  Gain=mParams.joints.hip.kStop
  Gain4 : Gain  Gain=1/mParams.joints.hip.wMaxStop
  Gain5 : Gain  Gain=-1
  Gain6 : Gain  Gain=-1
  Limit Joint Range : simulink/Logic and Bit Operations/Interval Test  Commented=on  IntervalClosedRight=on  uplimit=mParams.joints.hip.MaxPitch + 20*pi/180  IntervalClosedLeft=on  lowlimit=mParams.joints.hip.MinPitch - 20*pi/180  OutDataTypeStr=boolean
      settings: AttributesFormatString=|
      | Lower limits: %<lowlimit>
      | Upper limits: %<uplimit>
  Logical Operator3 : Logic  Commented=on  Operator=NOT  AllPortsSameDT=off  OutDataTypeStr=boolean
  Product1 : Product  Inputs=4
  Product2 : Product  Inputs=4
  Stop Simulation1 : Stop  Commented=on
  Sum : Sum  Inputs=|+-
  Sum1 : Sum  Inputs=|+-
  Sum2 : Sum
  Sum3 : Sum  Inputs=|-+
  Sum4 : Sum  Inputs=|-+
  above upper limit? : simulink/Logic and Bit Operations/Compare To Zero  relop=>  OutDataTypeStr=boolean  ZeroCross=off
  below lower limit? : simulink/Logic and Bit Operations/Compare To Zero  relop=<  OutDataTypeStr=boolean  ZeroCross=off
  const : Constant
  const1 : Constant
  mech limit pushes back? : simulink/Logic and Bit Operations/Compare To Zero  relop=>  OutDataTypeStr=boolean  ZeroCross=off
  mech limit pushes back?. : simulink/Logic and Bit Operations/Compare To Zero  relop=>  OutDataTypeStr=boolean  ZeroCross=off
  overextension angle : Constant  Value=mParams.joints.hip.MaxPitch
  overflexion angle : Constant  Value=mParams.joints.hip.MinPitch
  tau [Nm] : Outport  VectorParamsAs1DForOutWhenUnconnected=off
  wires:
  Gain5/1 -> Sum2/2
  Gain4/1 -> Gain2/1, Sum4/1
  const1/1 -> Sum4/2
  Sum4/1 -> Product2/3, mech limit pushes back?./1
  Gain1/1 -> below lower limit?/1, Product2/2
  mech limit pushes back?./1 -> Product2/4
  below lower limit?/1 -> Product2/1
  Product2/1 -> Gain5/1
  Product1/1 -> Gain6/1
  above upper limit?/1 -> Product1/1
  mech limit pushes back?/1 -> Product1/4
  Gain3/1 -> above upper limit?/1, Product1/2
  Sum3/1 -> mech limit pushes back?/1, Product1/3
  const/1 -> Sum3/2
  dq [rad/s]/1 -> Gain4/1
  overextension angle/1 -> Sum/2
  q [rad]/1 -> Limit Joint Range/1, Sum1/1, Sum/1
  Sum/1 -> Gain3/1
  Sum1/1 -> Gain1/1
  overflexion angle/1 -> Sum1/2
  Sum2/1 -> tau [Nm]/1
  Gain2/1 -> Sum3/1
  Gain6/1 -> Sum2/1
  Limit Joint Range/1 -> Logical Operator3/1
  Logical Operator3/1 -> Stop Simulation1/1

== system nmsRR/Body and Contact Model/L Leg/Hip Roll Mechanical Limits ==
  note: Overflexion Torque
  note: Joint Limits
  note: Overextension Torque
  dq [rad/s] : Inport
  q [rad] : Inport  Port=2
  Gain1 : Gain  Gain=mParams.joints.hip.kStop
  Gain2 : Gain  Gain=-1
  Gain3 : Gain  Gain=mParams.joints.hip.kStop
  Gain4 : Gain  Gain=1/mParams.joints.hip.wMaxStop
  Gain5 : Gain  Gain=-1
  Gain6 : Gain  Gain=-1
  Limit Joint Range : simulink/Logic and Bit Operations/Interval Test  Commented=on  IntervalClosedRight=on  uplimit=mParams.joints.hip.MaxRoll + 20*pi/180  IntervalClosedLeft=on  lowlimit=mParams.joints.hip.MinRoll - 20*pi/180  OutDataTypeStr=boolean
      settings: AttributesFormatString=|
      | Lower limits: %<lowlimit>
      | Upper limits: %<uplimit>
  Logical Operator3 : Logic  Commented=on  Operator=NOT  AllPortsSameDT=off  OutDataTypeStr=boolean
  Product1 : Product  Inputs=4
  Product2 : Product  Inputs=4
  Stop Simulation1 : Stop  Commented=on
  Sum : Sum  Inputs=|+-
  Sum1 : Sum  Inputs=|+-
  Sum2 : Sum
  Sum3 : Sum  Inputs=|-+
  Sum4 : Sum  Inputs=|-+
  above upper limit? : simulink/Logic and Bit Operations/Compare To Zero  relop=>  OutDataTypeStr=boolean  ZeroCross=off
  below lower limit? : simulink/Logic and Bit Operations/Compare To Zero  relop=<  OutDataTypeStr=boolean  ZeroCross=off
  const : Constant
  const1 : Constant
  mech limit pushes back? : simulink/Logic and Bit Operations/Compare To Zero  relop=>  OutDataTypeStr=boolean  ZeroCross=off
  mech limit pushes back?. : simulink/Logic and Bit Operations/Compare To Zero  relop=>  OutDataTypeStr=boolean  ZeroCross=off
  overextension angle : Constant  Value=mParams.joints.hip.MaxRoll
  overflexion angle : Constant  Value=mParams.joints.hip.MinRoll
  tau [Nm] : Outport  VectorParamsAs1DForOutWhenUnconnected=off
  wires:
  Gain5/1 -> Sum2/2
  Gain4/1 -> Gain2/1, Sum4/1
  const1/1 -> Sum4/2
  Sum4/1 -> Product2/3, mech limit pushes back?./1
  Gain1/1 -> below lower limit?/1, Product2/2
  mech limit pushes back?./1 -> Product2/4
  below lower limit?/1 -> Product2/1
  Product2/1 -> Gain5/1
  Product1/1 -> Gain6/1
  above upper limit?/1 -> Product1/1
  mech limit pushes back?/1 -> Product1/4
  Gain3/1 -> above upper limit?/1, Product1/2
  Sum3/1 -> mech limit pushes back?/1, Product1/3
  const/1 -> Sum3/2
  dq [rad/s]/1 -> Gain4/1
  overextension angle/1 -> Sum/2
  q [rad]/1 -> Limit Joint Range/1, Sum1/1, Sum/1
  Sum/1 -> Gain3/1
  Sum1/1 -> Gain1/1
  overflexion angle/1 -> Sum1/2
  Sum2/1 -> tau [Nm]/1
  Gain2/1 -> Sum3/1
  Gain6/1 -> Sum2/1
  Limit Joint Range/1 -> Logical Operator3/1
  Logical Operator3/1 -> Stop Simulation1/1

== system nmsRR/Body and Contact Model/L Leg/Knee Mechanical Limits ==
  note: Overflexion Torque
  note: Joint Limits
  note: Overextension Torque
  dq [rad/s] : Inport
  q [rad] : Inport  Port=2
  Gain1 : Gain  Gain=mParams.joints.knee.kStop
  Gain2 : Gain  Gain=-1
  Gain3 : Gain  Gain=mParams.joints.knee.kStop
  Gain4 : Gain  Gain=1/mParams.joints.knee.wMaxStop
  Gain5 : Gain  Gain=-1
  Gain6 : Gain  Gain=-1
  Limit Knee Range : simulink/Logic and Bit Operations/Interval Test  IntervalClosedRight=on  uplimit=mParams.joints.knee.MaxPitch + 20*pi/180  IntervalClosedLeft=on  lowlimit=mParams.joints.knee.MinPitch - 20*pi/180  OutDataTypeStr=boolean
      settings: AttributesFormatString=|
      | Lower limits: %<lowlimit>
      | Upper limits: %<uplimit>
  Logical Operator3 : Logic  Operator=NOT  AllPortsSameDT=off  OutDataTypeStr=boolean
  Product1 : Product  Inputs=4
  Product2 : Product  Inputs=4
  Stop Simulation1 : Stop
  Sum : Sum  Inputs=|+-
  Sum1 : Sum  Inputs=|+-
  Sum2 : Sum
  Sum3 : Sum  Inputs=|-+
  Sum4 : Sum  Inputs=|-+
  above upper limit? : simulink/Logic and Bit Operations/Compare To Zero  relop=>  OutDataTypeStr=boolean  ZeroCross=off
  below lower limit? : simulink/Logic and Bit Operations/Compare To Zero  relop=<  OutDataTypeStr=boolean  ZeroCross=off
  const : Constant
  const1 : Constant
  mech limit pushes back? : simulink/Logic and Bit Operations/Compare To Zero  relop=>  OutDataTypeStr=boolean  ZeroCross=off
  mech limit pushes back?. : simulink/Logic and Bit Operations/Compare To Zero  relop=>  OutDataTypeStr=boolean  ZeroCross=off
  overextension angle : Constant  Value=mParams.joints.knee.MaxPitch
  overflexion angle : Constant  Value=mParams.joints.knee.MinPitch
  tau [Nm] : Outport  VectorParamsAs1DForOutWhenUnconnected=off
  wires:
  Gain5/1 -> Sum2/2
  Gain4/1 -> Gain2/1, Sum4/1
  const1/1 -> Sum4/2
  Sum4/1 -> Product2/3, mech limit pushes back?./1
  Gain1/1 -> Product2/2, below lower limit?/1
  mech limit pushes back?./1 -> Product2/4
  below lower limit?/1 -> Product2/1
  Product2/1 -> Gain5/1
  Product1/1 -> Gain6/1
  above upper limit?/1 -> Product1/1
  mech limit pushes back?/1 -> Product1/4
  Gain3/1 -> above upper limit?/1, Product1/2
  Sum3/1 -> mech limit pushes back?/1, Product1/3
  const/1 -> Sum3/2
  dq [rad/s]/1 -> Gain4/1
  overextension angle/1 -> Sum/2
  q [rad]/1 -> Sum/1, Limit Knee Range/1, Sum1/1
  Sum/1 -> Gain3/1
  Sum1/1 -> Gain1/1
  overflexion angle/1 -> Sum1/2
  Sum2/1 -> tau [Nm]/1
  Gain2/1 -> Sum3/1
  Gain6/1 -> Sum2/1
  Limit Knee Range/1 -> Logical Operator3/1
  Logical Operator3/1 -> Stop Simulation1/1

== system nmsRR/Body and Contact Model/L Leg/Rotation Sensor Knee ==
  note: Rotation Sensor in World Frame
  Coordinate Transformation Conversion1 : robotcorelib/Coordinate Transformation Conversion  InputRepresentation=Quaternion  InputEulerSequence=ZYX  ShowTrVecInputPort=on  OutputRepresentation=Euler Angles  OutputEulerSequence=XYZ  ShowTrVecOutputPort=on  SimulateUsing=Code generation
      settings: SourceProductBaseCode=NV,RO,RR,UV
  Coordinate Transformation Conversion2 : robotcorelib/Coordinate Transformation Conversion  InputRepresentation=Quaternion  InputEulerSequence=ZYX  ShowTrVecInputPort=on  OutputRepresentation=Rotation Matrix  OutputEulerSequence=XYZ  ShowTrVecOutputPort=on  SimulateUsing=Code generation
      settings: SourceProductBaseCode=NV,RO,RR,UV
  Frame Sensor : sm_lib/Frames and Transforms/Transform Sensor  MeasurementFrame=World  SenseAngle=off  SenseAxis=off  SenseAngle1=off  SenseAngle2=off  SenseAngle3=off  SenseQ=on  SenseR=off  SenseOmegaX=off  SenseOmegaY=off  SenseOmegaZ=off  SenseOmega1=off  SenseOmega2=off  SenseOmega3=off  SenseQDot=off  SenseRDot=off  SenseAlphaX=off  SenseAlphaY=off  SenseAlphaZ=off  SenseAlpha1=off  SenseAlpha2=off  SenseAlpha3=off  SenseQDDot=off  SenseRDDot=off  SenseX=off  SenseY=off  SenseZ=off  SenseRad=off  SenseAzim=off  SenseDist=off  SenseInc=off  SenseXDot=off  SenseYDot=off  SenseZDot=off  SenseRadDot=off  SenseAzimDot=off  SenseDistDot=off  SenseIncDot=off  SenseXDDot=off  SenseYDDot=off  SenseZDDot=off  SenseRadDDot=off  SenseAzimDDot=off  SenseDistDDot=off  SenseIncDDot=off
  PS-Simulink Converter12 : nesl_utility/PS-Simulink Converter  PhysicalDomain=network_engine_domain  SubClassName=ps_output  LeftPortType=input  RightPortType=output  PseudoPeriodic=off  Frequencies=[]  Unit=1  AffineConversion=off
      settings: SourceProductBaseCode=PW,SS
  World Frame : sm_lib/Frames and Transforms/World Frame
  frame : PMIOPort  Side=Left
  rotation [rad] : Outport  VectorParamsAs1DForOutWhenUnconnected=off
  Rotation Matrix : Outport  Port=2  VectorParamsAs1DForOutWhenUnconnected=off
  wires:
  PS-Simulink Converter12/1 -> Coordinate Transformation Conversion2/1, Coordinate Transformation Conversion1/1
  Coordinate Transformation Conversion1/1 -> rotation [rad]/1
  Coordinate Transformation Conversion2/1 -> Rotation Matrix/1
  connections:
  Frame Sensor/RConn1 -- frame/RConn1
  World Frame/RConn1 -- Frame Sensor/LConn1
  PS-Simulink Converter12/LConn1 -- Frame Sensor/RConn2

== system nmsRR/Body and Contact Model/L Leg/Sensor Left Ankle ==
  note: Position and Velocity Sensor in World Frame
  Frame Sensor : sm_lib/Frames and Transforms/Transform Sensor  MeasurementFrame=Base  SenseAngle=off  SenseAxis=off  SenseAngle1=off  SenseAngle2=off  SenseAngle3=off  SenseQ=off  SenseR=off  SenseOmegaX=off  SenseOmegaY=off  SenseOmegaZ=off  SenseOmega1=off  SenseOmega2=off  SenseOmega3=off  SenseQDot=off  SenseRDot=off  SenseAlphaX=off  SenseAlphaY=off  SenseAlphaZ=off  SenseAlpha1=off  SenseAlpha2=off  SenseAlpha3=off  SenseQDDot=off  SenseRDDot=off  SenseX=on  SenseY=on  SenseZ=on  SenseRad=off  SenseAzim=off  SenseDist=off  SenseInc=off  SenseXDot=on  SenseYDot=on  SenseZDot=on  SenseRadDot=off  SenseAzimDot=off  SenseDistDot=off  SenseIncDot=off  SenseXDDot=off  SenseYDDot=off  SenseZDDot=off  SenseRadDDot=off  SenseAzimDDot=off  SenseDistDDot=off  SenseIncDDot=off
  Mux : Mux  Inputs=3
  Mux1 : Mux  Inputs=3
  PS-Simulink Converter1 : nesl_utility/PS-Simulink Converter  PhysicalDomain=network_engine_domain  SubClassName=ps_output  LeftPortType=input  RightPortType=output  PseudoPeriodic=off  Frequencies=[]  Unit=m  AffineConversion=off
      settings: SourceProductBaseCode=PW,SS
  PS-Simulink Converter12 : nesl_utility/PS-Simulink Converter  PhysicalDomain=network_engine_domain  SubClassName=ps_output  LeftPortType=input  RightPortType=output  PseudoPeriodic=off  Frequencies=[]  Unit=m  AffineConversion=off
      settings: SourceProductBaseCode=PW,SS
  PS-Simulink Converter2 : nesl_utility/PS-Simulink Converter  PhysicalDomain=network_engine_domain  SubClassName=ps_output  LeftPortType=input  RightPortType=output  PseudoPeriodic=off  Frequencies=[]  Unit=m  AffineConversion=off
      settings: SourceProductBaseCode=PW,SS
  PS-Simulink Converter3 : nesl_utility/PS-Simulink Converter  PhysicalDomain=network_engine_domain  SubClassName=ps_output  LeftPortType=input  RightPortType=output  PseudoPeriodic=off  Frequencies=[]  Unit=m/s  AffineConversion=off
      settings: SourceProductBaseCode=PW,SS
  PS-Simulink Converter4 : nesl_utility/PS-Simulink Converter  PhysicalDomain=network_engine_domain  SubClassName=ps_output  LeftPortType=input  RightPortType=output  PseudoPeriodic=off  Frequencies=[]  Unit=m/s  AffineConversion=off
      settings: SourceProductBaseCode=PW,SS
  PS-Simulink Converter5 : nesl_utility/PS-Simulink Converter  PhysicalDomain=network_engine_domain  SubClassName=ps_output  LeftPortType=input  RightPortType=output  PseudoPeriodic=off  Frequencies=[]  Unit=m/s  AffineConversion=off
      settings: SourceProductBaseCode=PW,SS
  World Frame : sm_lib/Frames and Transforms/World Frame
  Frame : PMIOPort  Side=Left
  Position [m] : Outport  VectorParamsAs1DForOutWhenUnconnected=off
  Velocity [m/s] : Outport  Port=2  VectorParamsAs1DForOutWhenUnconnected=off
  wires:
  PS-Simulink Converter12/1 -> Mux/1
  PS-Simulink Converter1/1 -> Mux/2
  PS-Simulink Converter2/1 -> Mux/3
  Mux/1 -> Position [m]/1
  PS-Simulink Converter5/1 -> Mux1/3
  PS-Simulink Converter4/1 -> Mux1/1
  Mux1/1 -> Velocity [m/s]/1
  PS-Simulink Converter3/1 -> Mux1/2
  connections:
  Frame Sensor/RConn1 -- Frame/RConn1
  PS-Simulink Converter12/LConn1 -- Frame Sensor/RConn2
  Frame Sensor/RConn3 -- PS-Simulink Converter1/LConn1
  Frame Sensor/RConn4 -- PS-Simulink Converter2/LConn1
  Frame Sensor/RConn7 -- PS-Simulink Converter5/LConn1
  Frame Sensor/RConn5 -- PS-Simulink Converter4/LConn1
  Frame Sensor/RConn6 -- PS-Simulink Converter3/LConn1
  World Frame/RConn1 -- Frame Sensor/LConn1

== system nmsRR/Body and Contact Model/L Leg/Shank ==
  Solid : sm_lib/Body Elements/Brick Solid  GraphicAmbientColor=[0.15 0.15 0.15 1.0]  BasedOnType=Density  BrickDimensions="[mParams.bodies.shank.d  mParams.bodies.shank.l mParams.bodies.shank.b]"  BrickDimensionUnits=m  CenterOfMass=mParams.bodies.shank.CG  CenterOfMassUnits=m  GraphicDiffuseColor=[1 0.5 0.5]  Density=2.7  DensityUnits=g/cm^3  DoExposeReferenceFrame=on  GraphicEmissiveColor=[0 0 0 1.0]  ExportEntireGeometry=off  SerializedFrames=<Frames><Frame><Id>Frame1</Id><Value><Name>F1</Name><Origin><Source>CenterOfMassFrame</Source><FeatureName></FeatureName></Origin><PrimaryAxis><DefinedDirection>+Z</DefinedDirection><Source>ReferenceFrame</Source><SourceDirection>+Z</SourceDirection><FeatureName></FeatureName></PrimaryAxis><SecondaryAxis><DefinedDirection>+X</DefinedDirection><Source>ReferenceFrame</Source><SourceDirection>+X</SourceDirection><FeatureName></FeatureName></SecondaryAxis></Value></Frame></Frames>  MarkerShape=Sphere  MarkerSize=10  GraphicType=FromGeometry  InertiaType=Custom  Mass=mParams.bodies.shank.m  MassUnits=kg  MomentsOfInertia=mParams.bodies.shank.In  MomentsOfInertiaUnits=kg*m^2  GraphicOpacity=1.0  ProductsOfInertia=[0 0 0]  ProductsOfInertiaUnits=kg*m^2  GraphicShininess=75  GraphicSpecularColor=[0.5 0.5 0.5 1.0]  GraphicVisPropType=SimpleVisualProperties
  Transform CS1 to MidSegment : sm_lib/Frames and Transforms/Rigid Transform  TranslationMethod=Cartesian  TranslationStandardOffset=0  TranslationLengthUnit=m  TranslationStandardAxis=+Y  TranslationCartesianOffset=[0 -mParams.bodies.shank.l/2 0]  TranslationROffset=0  TranslationROffsetUnits=m  TranslationZOffset=0  TranslationZOffsetUnits=m  TranslationThetaOffset=0  TranslationThetaOffsetUnits=deg  RotationMethod=None  RotationAngleUnits=deg  RotationStandardAxis=+X  RotationAngle=-90  RotationArbitraryAxis=[0 0 1]  FollAlignAxisA=+X  BaseAlignAxisA=+Y  FollAlignAxisB=+Y  BaseAlignAxisB=+Z  RotationSequenceAxes=FollowerAxes  RotationSequence=XYX  RotationSequenceAngles=[0 0 0]  RotationSequenceAnglesUnits=deg  RotationMatrix=[1 0 0; 0 1 0; 0 0 1]
  Transform MidSegment to CS2 : sm_lib/Frames and Transforms/Rigid Transform  TranslationMethod=Cartesian  TranslationStandardOffset=0  TranslationLengthUnit=m  TranslationStandardAxis=+Y  TranslationCartesianOffset=[ 0 -mParams.bodies.shank.l/2 0]  TranslationROffset=0  TranslationROffsetUnits=m  TranslationZOffset=0  TranslationZOffsetUnits=m  TranslationThetaOffset=0  TranslationThetaOffsetUnits=deg  RotationMethod=None  RotationAngleUnits=deg  RotationStandardAxis=+X  RotationAngle=90  RotationArbitraryAxis=[0 0 1]  FollAlignAxisA=+X  BaseAlignAxisA=+Y  FollAlignAxisB=+Y  BaseAlignAxisB=+Z  RotationSequenceAxes=FollowerAxes  RotationSequence=XYX  RotationSequenceAngles=[0 0 0]  RotationSequenceAnglesUnits=deg  RotationMatrix=[1 0 0; 0 1 0; 0 0 1]
  CS1 : PMIOPort  Side=Left
  CS2 : PMIOPort  Port=2  Side=Right
  connections:
  Transform MidSegment to CS2/RConn1 -- CS2/RConn1
  Transform CS1 to MidSegment/LConn1 -- CS1/RConn1
  Solid/RConn1 -- Transform CS1 to MidSegment/RConn1 -- Transform MidSegment to CS2/LConn1
